simulink model "Practica_2"  (R2012b)
settings: Solver=ode45  StartTime=0.0  StopTime=20.0  RelTol=1e-3
values from neighbouring files (symbols this model uses):
  B = [12 3 1 0; 0 1 0 5; 0 0 5 7; 0 0 0 1]    [Ejercicio2.m]    (also in Poligonos.m = [A;ones(1,k)]; refleja.m = [A;ones(1,k)])
  M = solve([H(1)==0,H(2)==0,H(3)==0,H(4)==0],[x,y,z,t])    [Ejercicio2.m]    (also in Poligonos.m = [N,v]; esferica.m = [u1' u2' u3']; refleja.m = [N,v])
undefined symbols (not defined in the file or in its folder): K
settings Model: Creator=isa  LastModifiedBy=isa

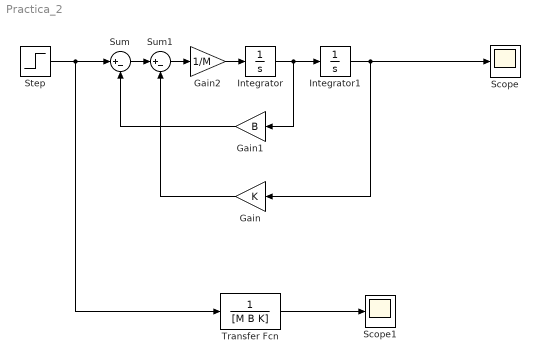
== system Practica_2 ==
  Gain : Gain  Gain=K
  Gain1 : Gain  Gain=B
  Gain2 : Gain  Gain=1/M
  Integrator : Integrator
  Integrator1 : Integrator
  Scope : Scope
      settings: TimeRange=4  YMin=-0.2812499999999998  YMax=2.11875
  Scope1 : Scope
  Step : Step  SampleTime=0
  Sum : Sum  Inputs=|+-
  Sum1 : Sum  Inputs=|+-
  Transfer Fcn : TransferFcn  Denominator=[M B K]
  wires:
  Integrator/1 -> Gain1/1, Integrator1/1
  Integrator1/1 -> Gain/1, Scope/1
  Step/1 -> Transfer Fcn/1, Sum/1
  Gain1/1 -> Sum/2
  Sum/1 -> Sum1/1
  Gain/1 -> Sum1/2
  Gain2/1 -> Integrator/1
  Sum1/1 -> Gain2/1
  Transfer Fcn/1 -> Scope1/1
